simulink model "symolinc1"  (R2018b)
settings: Solver=VariableStepAuto  StartTime=0.0  StopTime=10.0  RelTol=1e-3
libraries: dspsrcs4 x1
settings Model: Creator=Sazgar Shargh  LastModifiedBy=Sazgar Shargh

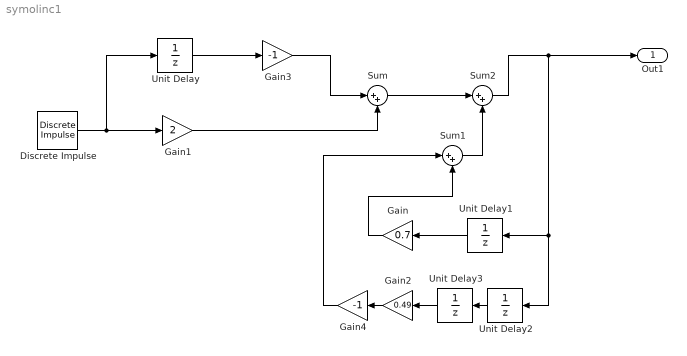
== system symolinc1 ==
  Discrete Impulse : dspsrcs4/Discrete  Impulse  Delay=0  SampleTime=1  FrameSample=1  OutputFrames=off  dataType=double  isSigned=on  wordLen=16  udDataType=sfix(16)  fracBitsMode=Best precision  numFracBits=15  OutDataTypeStr=double  LastOutDataTypeStr=double
  Gain : Gain  Gain=0.7
  Gain1 : Gain  Gain=2
  Gain2 : Gain  Gain=0.49
  Gain3 : Gain  Gain=-1
  Gain4 : Gain  Gain=-1
  Sum : Sum  Inputs=|++
  Sum1 : Sum  Inputs=|++
  Sum2 : Sum  Inputs=|++
  Unit Delay{,1..3} (4 alike) : UnitDelay  SampleTime=-1
  Out1 : Outport  SignalName=11
  wires:
  Discrete Impulse/1 -> Unit Delay/1, Gain1/1
  Unit Delay/1 -> Gain3/1
  Gain3/1 -> Sum/1
  Gain1/1 -> Sum/2
  Sum/1 -> Sum2/1
  Sum1/1 -> Sum2/2
  Sum2/1 -> Out1/1, Unit Delay2/1, Unit Delay1/1
  Unit Delay1/1 -> Gain/1
  Gain/1 -> Sum1/2
  Unit Delay2/1 -> Unit Delay3/1
  Unit Delay3/1 -> Gain2/1
  Gain2/1 -> Gain4/1
  Gain4/1 -> Sum1/1
